simulink library "transformations_lib"  (R2015b)
settings: Solver=VariableStepAuto  StartTime=0.0  StopTime=10.0  RelTol=1e-3
settings Model: Creator=zachn  LastModifiedBy=zachn

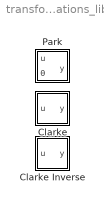
== system transformations_lib ==
  Clarke : Subsystem
      mask init:
      | p_mat = (2/3) * [   1       -1/2        -1/2; 
      |                     0       sqrt(3)/2   -sqrt(3)/2;
      |                     1/2     1/2         1/2
      |                 ];
      mask DialogControl DescGroupVar Prompt: Clarke Transformation
      mask Display:
      | % fprintf('P');
      | 
      | text(0.55,0.55,'P','horizontalAlignment','center','verticalAlignment','middle','texmode','on');
  Clarke Inverse : Subsystem
      mask init:
      | p_mat = (2/3) * [   1       -1/2        -1/2; 
      |                     0       sqrt(3)/2   -sqrt(3)/2;
      |                     1/2     1/2         1/2
      |                 ];
      | p_inv = inv(p_mat);
      mask DialogControl DescGroupVar Prompt: Inverse Clarke Transformation
      mask DialogControl DescTextVar Prompt: Clarke transformation matrix for translating back from a 2-phase representation to 3-phases.
      mask DialogControl Control2 Prompt: y = P^(-1).*u
      mask Display: text(0.55,0.55,'P^{-1}','horizontalAlignment','center','verticalAlignment','middle','texmode','on');
  Park : Subsystem  mask{IsInverse=off}
      mask prompts: IsInverse "Inverse"
      mask init:
      | is_inverse = 0;
      | 
      | param = get_param(gcb, 'IsInverse');
      | 
      | if strcmp(param, 'on')
      |     is_inverse = 1;
      | else
      |     is_inverse = 0;
      | end
      mask DialogControl DescGroupVar Prompt: Park Transformation
      mask DialogControl Container4 Prompt: Main
      mask Display:
      | % fprintf('P');
      | fprintf('');
      | 
      | param = get_param(gcb, 'IsInverse');
      | 
      | if strcmp(param, 'on')
      |     text(0.55,0.75,'T(\theta)^{-1}','horizontalAlignment','center','verticalAlignment','middle','Interpreter','tex');
      | else
      |     text(0.55,0.65,'T(\theta)','horizontalAlignment','center','verticalAlignment','middle','Interpreter','tex');
      | end
      | 
      | port_label('input',2,'\angle','Interpreter','tex');

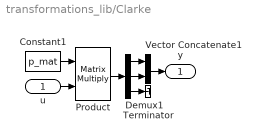
== system transformations_lib/Clarke ==
  u : Inport
  Constant1 : Constant  Value=p_mat  VectorParams1D=off
  Demux1 : Demux  Outputs=3
  Product : Product  Multiplication=Matrix(*)
  Terminator : Terminator
  Vector Concatenate1 : Concatenate  Mode=Multidimensional array
  y : Outport
  wires:
  Constant1/1 -> Product/1
  u/1 -> Product/2
  Demux1/2 -> Vector Concatenate1/2
  Demux1/1 -> Vector Concatenate1/1
  Demux1/3 -> Terminator/1
  Vector Concatenate1/1 -> y/1
  Product/1 -> Demux1/1

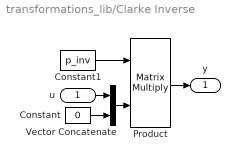
== system transformations_lib/Clarke Inverse ==
  u : Inport
  Constant : Constant  Value=0  VectorParams1D=off
  Constant1 : Constant  Value=p_inv  VectorParams1D=off
  Product : Product  Multiplication=Matrix(*)
  Vector Concatenate : Concatenate  Mode=Multidimensional array
  y : Outport
  wires:
  Constant/1 -> Vector Concatenate/2
  u/1 -> Vector Concatenate/1
  Constant1/1 -> Product/1
  Vector Concatenate/1 -> Product/2
  Product/1 -> y/1

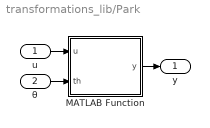
== system transformations_lib/Park ==
  u : Inport
  θ : Inport  Port=2
  MATLAB Function : MATLAB Function  TreatAsAtomicUnit=on  mask{inverse=is_inverse}
      mask prompts: inverse "Take Inverse"
  y : Outport
  wires:
  u/1 -> MATLAB Function/1(u)
  θ/1 -> MATLAB Function/2(th)
  MATLAB Function/1(y) -> y/1

== matlab function transformations_lib/Park/MATLAB Function ==
  data: u input; th input; y output; inverse parameter
function y = t_mult(u, th, inverse)

if inverse > 0
    th = -th; 
end

T = [	cos(th)	-sin(th)	;
        sin(th)	 cos(th)	];


y = T*u;
